simulink library "Steer_Ackermann_WheelsOnly"  (R2023a)
settings: Solver=VariableStepAuto  StartTime=0.0  StopTime=10.0  RelTol=1e-3
undefined symbols (not defined in the file): Steer, X, Y, Z
libraries: sm_lib x2, Suspension_Utilities x2, nesl_utility x2, Body_Utilities x1, Steer_Control_Axle2 x1
Description:
  | Component of Simscape Vehicle Templates Library
  | 
  | Copyright 2018-2024 The MathWorks, Inc.
settings Model: Creator=smiller  LastModifiedBy=smiller
settings SolverCC: AlgebraicLoopSolver=TrustRegion
settings DataIOCC: ReturnWorkspaceOutputs=off
settings DebuggingCC: UnconnectedInputMsg=warning  UnconnectedOutputMsg=warning  UnconnectedLineMsg=warning  ArithmeticOperatorsInVariantConditions=warning
settings ModelReferenceCC: EnableRefExpFcnMdlSchedulingChecks=on
settings SFSimCC: CustomCodeUndefinedFunction=UseInterfaceOnly
settings RTWCC: DLArmComputeVersion=19.05

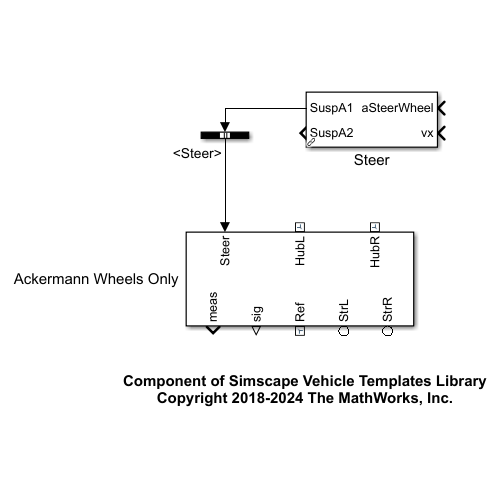
[thumbnail: Simulink's stored preview of the top-level diagram]
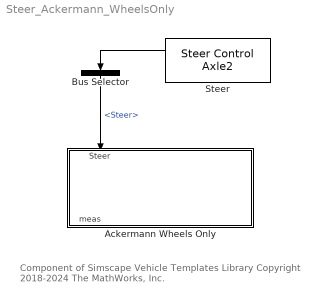
== system Steer_Ackermann_WheelsOnly ==
  note: Component of Simscape Vehicle Templates Library
      | Copyright 2018-2024 The MathWorks, Inc.
  Ackermann Wheels Only : Subsystem  VariantControl=Ackermann  mask(Ackerman Steering, Wheels only){whl2rack_filter=1/Steer.Rack.fActuatorCutoff.Value, yTrack=Steer.xTrack.Value, xwheelbase=Steer.xWheelbase.Value, steer_ratio=Steer.rSteer.Value, aCaster=Steer.aCaster.Value, aKPI=Steer.aKPI.Value}
      mask prompts: whl2rack_filter "Rack Motion Filter (sec)"; yTrack "Track Width (m)"; xwheelbase "Wheelbase (m)"; steer_ratio "Steer Ratio"; aCaster "Caster Angle (deg)"; aKPI "King Pin Inclination (KPI) Angle (deg)"
      mask help: Converts commanded steering wheel angle to wheel steer angle using steering ratio parameters and function. Steering wheel not shown in animation.
      mask TypeOptions aCaster:
      | Revolute
      | SteerL/aCaster | Revolute
      | SteerR/aCaster
      mask TypeOptions aKPI:
      | Revolute
      | SteerL/aKPI | Revolute
      | SteerR/aKPI
      mask DialogControl cont_steer Prompt: Steer
  Bus Selector : BusSelector  OutputSignals=Steer
  Steer : Steer_Control_Axle2/Steer Control Axle2  Steer=Control.Default.Steer
  wires:
  Steer/1 -> Bus Selector/1
  Bus Selector/1 -> Ackermann Wheels Only/1(Steer)  "<Steer>"

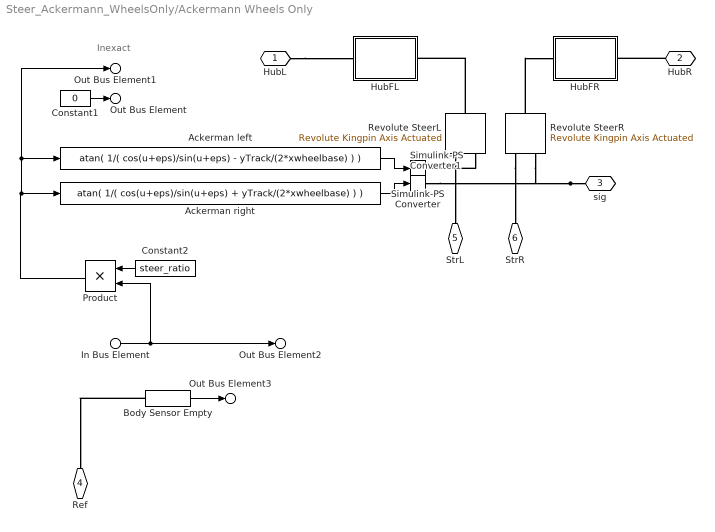
== system Steer_Ackermann_WheelsOnly/Ackermann Wheels Only ==
  note: Inexact
  In Bus Element : Inport  PortName=Steer  Element=aSteerWheel
  Ackerman left : Fcn  Expr=atan( 1/( cos(u+eps)/sin(u+eps) - yTrack/(2*xwheelbase) ) )
  Ackerman right : Fcn  Expr=atan( 1/( cos(u+eps)/sin(u+eps) + yTrack/(2*xwheelbase) ) )
  Body Sensor Empty : Body_Utilities/Body Sensor Empty  offset_body_sensor=Vehicle.Chassis.Body.sCG.Value
  Constant1 : Constant  Value=0
  Constant2 : Constant  Value=steer_ratio
  HubFL : Subsystem
  HubFR : Subsystem
  Product : Product
  Revolute SteerL : Suspension_Utilities/Revolute Kingpin Axis Actuated  popup_leftRight=Left  aCaster=aCaster  aKPI=aKPI
  Revolute SteerR : Suspension_Utilities/Revolute Kingpin Axis Actuated  popup_leftRight=Right  aCaster=aCaster  aKPI=aKPI
  Simulink-PS Converter : nesl_utility/Simulink-PS Converter  PhysicalDomain=network_engine_domain  SubClassName=ps_input  LeftPortType=input  RightPortType=output  PseudoPeriodic=off  Frequencies=[]  NoiseDistribution=none  NoiseParameters=[]  Unit=rad  AffineConversion=off  FilteringAndDerivatives=filter  SimscapeFilterOrder=2  InputFilterTimeConstant=whl2rack_filter  UdotUserProvided=0
  Simulink-PS Converter1 : nesl_utility/Simulink-PS Converter  PhysicalDomain=network_engine_domain  SubClassName=ps_input  LeftPortType=input  RightPortType=output  PseudoPeriodic=off  Frequencies=[]  NoiseDistribution=none  NoiseParameters=[]  Unit=rad  AffineConversion=off  FilteringAndDerivatives=filter  SimscapeFilterOrder=2  InputFilterTimeConstant=whl2rack_filter  UdotUserProvided=0
  HubL : PMIOPort  Side=Left
  HubR : PMIOPort  Port=2  Side=Left
  sig : PMIOPort  Port=3  Side=Right
  Ref : PMIOPort  Port=4  Side=Right
  StrL : PMIOPort  Port=5  Side=Right
  StrR : PMIOPort  Port=6  Side=Right
  Out Bus Element2 : Outport  VectorParamsAs1DForOutWhenUnconnected=off  PortName=meas  Element=aWheel
  Out Bus Element3 : Outport  VectorParamsAs1DForOutWhenUnconnected=off  PortName=meas  Element=Driver
  Out Bus Element : Outport  VectorParamsAs1DForOutWhenUnconnected=off  PortName=meas  Element=FRack
  Out Bus Element1 : Outport  VectorParamsAs1DForOutWhenUnconnected=off  PortName=meas  Element=xRack
  wires:
  Ackerman left/1 -> Simulink-PS Converter/1
  Ackerman right/1 -> Simulink-PS Converter1/1
  In Bus Element/1 -> Product/2, Out Bus Element2/1
  Body Sensor Empty/1 -> Out Bus Element3/1
  Constant1/1 -> Out Bus Element/1
  Product/1 -> Out Bus Element1/1, Ackerman left/1, Ackerman right/1
  Constant2/1 -> Product/1
  connections:
  HubL/RConn1 -- HubFL/RConn1
  Revolute SteerL/LConn1 -- StrL/RConn1
  Revolute SteerL/LConn2 -- Simulink-PS Converter/RConn1
  Revolute SteerL/RConn1 -- HubFL/LConn1
  Revolute SteerR/LConn1 -- StrR/RConn1
  Revolute SteerR/RConn1 -- HubFR/LConn1
  sig/RConn1 -- Revolute SteerR/LConn2 -- Simulink-PS Converter1/RConn1
  HubR/RConn1 -- HubFR/RConn1
  Body Sensor Empty/LConn1 -- Ref/RConn1

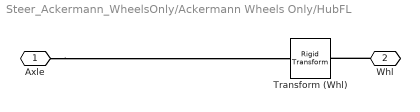
== system Steer_Ackermann_WheelsOnly/Ackermann Wheels Only/HubFL ==
  Transform (Whl) : sm_lib/Frames and Transforms/Rigid Transform  TranslationMethod=None  TranslationStandardOffset=0  TranslationStandardOffsetUnits=m  TranslationStandardAxis=+Z  TranslationCartesianOffset=[0 0 0]  TranslationCartesianOffsetUnits=m  TranslationROffset=0  TranslationROffsetUnits=m  TranslationZOffset=0  TranslationZOffsetUnits=m  TranslationThetaOffset=0  TranslationThetaOffsetUnits=deg  RotationMethod=StandardAxis  RotationAngleUnits=deg  RotationStandardAxis=-X  RotationAngle=90  RotationArbitraryAxis=[0 0 1]  FollAlignAxisA=+X  BaseAlignAxisA=+Y  FollAlignAxisB=+Y  BaseAlignAxisB=+Z  RotationSequenceAxes=FollowerAxes  RotationSequence=XYX  RotationSequenceAngles=[0 0 0]  RotationSequenceAnglesUnits=deg  RotationMatrix=[1 0 0; 0 1 0; 0 0 1]  Quaternion=[1 0 0 0]
  Axle : PMIOPort  Side=Left
  Whl : PMIOPort  Port=2  Side=Right
  connections:
  Whl/RConn1 -- Transform (Whl)/RConn1
  Axle/RConn1 -- Transform (Whl)/LConn1

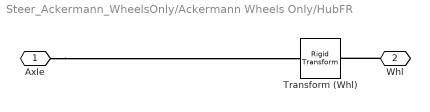
== system Steer_Ackermann_WheelsOnly/Ackermann Wheels Only/HubFR ==
  Transform (Whl) : sm_lib/Frames and Transforms/Rigid Transform  TranslationMethod=None  TranslationStandardOffset=0  TranslationStandardOffsetUnits=m  TranslationStandardAxis=+Z  TranslationCartesianOffset=[0 0 0]  TranslationCartesianOffsetUnits=m  TranslationROffset=0  TranslationROffsetUnits=m  TranslationZOffset=0  TranslationZOffsetUnits=m  TranslationThetaOffset=0  TranslationThetaOffsetUnits=deg  RotationMethod=StandardAxis  RotationAngleUnits=deg  RotationStandardAxis=-X  RotationAngle=90  RotationArbitraryAxis=[0 0 1]  FollAlignAxisA=+X  BaseAlignAxisA=+Y  FollAlignAxisB=+Y  BaseAlignAxisB=+Z  RotationSequenceAxes=FollowerAxes  RotationSequence=XYX  RotationSequenceAngles=[0 0 0]  RotationSequenceAnglesUnits=deg  RotationMatrix=[1 0 0; 0 1 0; 0 0 1]  Quaternion=[1 0 0 0]
  Axle : PMIOPort  Side=Left
  Whl : PMIOPort  Port=2  Side=Right
  connections:
  Whl/RConn1 -- Transform (Whl)/RConn1
  Axle/RConn1 -- Transform (Whl)/LConn1
